simulink model "Rasmusson"  (Simulink 7.1)
settings: Solver=ode15s  StartTime=0.0  StopTime=500  FixedStep=1e-4  MaxStep=0.1  RelTol=1e-6
undefined symbols (not defined in the file): Acap, aKss, ato_f, ato_s, aur, C2, C3, C4, Cai, CaJSR, CaNSR, Cao, Cass, CK1, CK2, Cm, CMDN_tot, CNa1, CNa2, CSQN_tot, ECa_L, ECl, F, GCab, GCaL, GCl_Ca, GKr, GKs, GKss, GKtof, GKtos, GKur, GNa, GNab, HTRPN_tot, HTRPNCa, I1, I1Na, I2, I2Na, I3, ICaL_max, ICNa2, ICNa3, IFNa, IK, iKss, INaK_max, Ip_Ca_max, ito_f, ito_s, iur, ka1, ka2, kb, kb1, kb2, kc1, kc2, kf ... (+45)
(part 2 of 2)

== system Rasmusson/Concentrations/Caconcentration/Cafluxes/Jtrpn ==
  Add : Sum  Inputs=+-+-  OutDataType=sfix(16)  OutScaling=2^-10
  Divide : Product  Inputs=***  OutDataType=sfix(16)  OutScaling=2^-10
  Divide1 : Product  Inputs=**  OutDataType=sfix(16)  OutScaling=2^-10
  Divide2 : Product  Inputs=***  OutDataType=sfix(16)  OutScaling=2^-10
  Divide3 : Product  Inputs=**  OutDataType=sfix(16)  OutScaling=2^-10
  HTRPNtot : Constant  Value=HTRPN_tot  OutDataType=sfix(16)  OutScaling=2^0
  LTRPNtot : Constant  Value=LTRPN_tot  OutDataType=sfix(16)  OutScaling=2^0
  Subtract : Sum  Inputs=+-  OutDataType=sfix(16)  OutScaling=2^-10
  Subtract1 : Sum  Inputs=+-  OutDataType=sfix(16)  OutScaling=2^-10
  khtrpn+ : Constant  Value=khtrpn1  OutDataType=sfix(16)  OutScaling=2^0
  khtrpn- : Constant  Value=khtrpn2  OutDataType=sfix(16)  OutScaling=2^0
  kltrpn+ : Constant  Value=kltrpn1  OutDataType=sfix(16)  OutScaling=2^0
  kltrpn- : Constant  Value=kltrpn2  OutDataType=sfix(16)  OutScaling=2^0
  tag scope: Jtrpn=global
  wires:
  Add/1 -> [Jtrpn]
  Divide/1 -> Add/1
  khtrpn+/1 -> Divide/1
  [Cai] -> Divide/2, Divide2/2
  Subtract/1 -> Divide/3
  HTRPNtot/1 -> Subtract/1
  [HTRPNCa] -> Subtract/2, Divide1/2
  Divide1/1 -> Add/2
  khtrpn-/1 -> Divide1/1
  Divide2/1 -> Add/3
  kltrpn+/1 -> Divide2/1
  Subtract1/1 -> Divide2/3
  LTRPNtot/1 -> Subtract1/1
  [LTRPNCa] -> Subtract1/2, Divide3/2
  Divide3/1 -> Add/4
  kltrpn-/1 -> Divide3/1

== system Rasmusson/Concentrations/Caconcentration/Cafluxes/Jup ==
  Add : Sum  OutDataType=sfix(16)  OutScaling=2^-10
  Divide : Product  Inputs=**/  OutDataType=sfix(16)  OutScaling=2^-10
  Kmup : Constant  Value=Km_up  OutDataType=sfix(16)  OutScaling=2^0
  Product : Product  OutDataType=sfix(16)  OutScaling=2^0  RndMeth=Zero
  Product1 : Product  OutDataType=sfix(16)  OutScaling=2^0  RndMeth=Zero
  nu3 : Constant  Value=nu3  OutDataType=sfix(16)  OutScaling=2^0
  tag scope: Jup=global
  wires:
  Divide/1 -> [Jup]
  nu3/1 -> Divide/1
  [Cai] -> Product/1, Product/2
  Product/1 -> Divide/2, Add/1
  Add/1 -> Divide/3
  Kmup/1 -> Product1/1, Product1/2
  Product1/1 -> Add/2

== system Rasmusson/Concentrations/Caconcentration/Cafluxes/Jxfer ==
  Divide : Product  Inputs=*/  OutDataType=sfix(16)  OutScaling=2^-10
  Subtract : Sum  Inputs=+-  OutDataType=sfix(16)  OutScaling=2^-10
  tauxfer : Constant  Value=tauxfer  OutDataType=sfix(16)  OutScaling=2^0
  tag scope: Jxfer=global
  wires:
  Divide/1 -> [Jxfer]
  [Cass] -> Subtract/1
  [Cai] -> Subtract/2
  tauxfer/1 -> Divide/2
  Subtract/1 -> Divide/1

== system Rasmusson/Concentrations/Caconcentration/Cafluxes/PRyR ==
  Add : Sum  OutDataType=sfix(16)  OutScaling=2^-10
  Divide : Product  Inputs=**/  OutDataType=sfix(16)  OutScaling=2^-10
  Fcn : Fcn  Expr=exp(-(u-5)*(u-5)/648)
  Gain : Gain  Gain=-0.04  ParameterDataType=sfix(16)  ParameterScaling=2^0  OutDataType=sfix(16)  OutScaling=2^0
  Gain1 : Gain  Gain=-0.1  ParameterDataType=sfix(16)  ParameterScaling=2^0  OutDataType=sfix(16)  OutScaling=2^0
  ICaLmax : Constant  Value=ICaL_max  OutDataType=sfix(16)  OutScaling=2^0
  Integrator : Integrator  InitialConditionSource=external
  PRyR : Constant  Value=PRyR  OutDataType=sfix(16)  OutScaling=2^0
  tag scope: PRyR=global
  wires:
  Integrator/1 -> [PRyR], Gain/1
  Add/1 -> Integrator/1
  [ICAL] -> Divide/1
  Fcn/1 -> Divide/2
  ICaLmax/1 -> Divide/3
  [volt] -> Fcn/1
  Divide/1 -> Gain1/1
  Gain1/1 -> Add/2
  Gain/1 -> Add/1
  PRyR/1 -> Integrator/2

== system Rasmusson/Concentrations/Caconcentration/Ryanodine_receptors/PC1 ==
  Constant : Constant  OutDataType=sfix(16)  OutScaling=2^0
  Subtract : Sum  Inputs=+---  OutDataType=sfix(16)  OutScaling=2^-10
  tag scope: PC1=global
  wires:
  Subtract/1 -> [PC1]
  Constant/1 -> Subtract/1
  [PC2] -> Subtract/2
  [PO1] -> Subtract/3
  [PO2] -> Subtract/4

== system Rasmusson/Concentrations/Caconcentration/Ryanodine_receptors/PC2 ==
  Integrator : Integrator  InitialConditionSource=external  InitialCondition=0.16774e-3
  PC2 : Constant  Value=PC2  OutDataType=sfix(16)  OutScaling=2^0
  Product : Product  OutDataType=sfix(16)  OutScaling=2^0  RndMeth=Zero
  Product1 : Product  OutDataType=sfix(16)  OutScaling=2^0  RndMeth=Zero
  Subtract : Sum  Inputs=+-  OutDataType=sfix(16)  OutScaling=2^-10
  kc+ : Constant  Value=kc1  OutDataType=sfix(16)  OutScaling=2^0
  kc- : Constant  Value=kc2  OutDataType=sfix(16)  OutScaling=2^0
  tag scope: PC2=global
  wires:
  kc-/1 -> Product1/1
  kc+/1 -> Product/1
  Product1/1 -> Subtract/2
  Product/1 -> Subtract/1
  Integrator/1 -> Product1/2, [PC2]
  Subtract/1 -> Integrator/1
  [PO1] -> Product/2
  PC2/1 -> Integrator/2

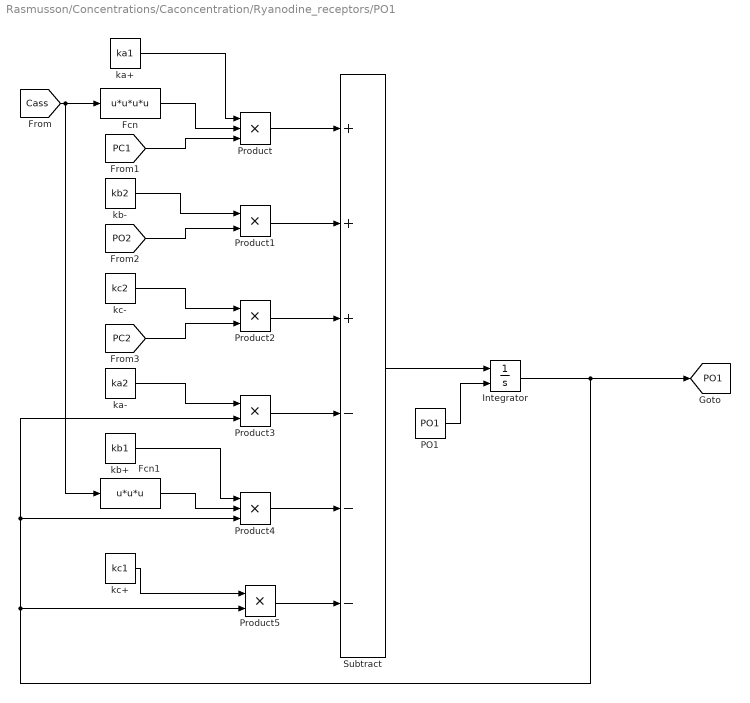
== system Rasmusson/Concentrations/Caconcentration/Ryanodine_receptors/PO1 ==
  Fcn : Fcn  Expr=u*u*u*u
  Fcn1 : Fcn  Expr=u*u*u
  Integrator : Integrator  InitialConditionSource=external  InitialCondition=0.149102e-4
  PO1 : Constant  Value=PO1  OutDataType=sfix(16)  OutScaling=2^0
  Product : Product  Inputs=3  OutDataType=sfix(16)  OutScaling=2^0  RndMeth=Zero
  Product{1..3,5} (4 alike) : Product  OutDataType=sfix(16)  OutScaling=2^0  RndMeth=Zero
  Product4 : Product  Inputs=3  OutDataType=sfix(16)  OutScaling=2^0  RndMeth=Zero
  Subtract : Sum  Inputs=+++---  OutDataType=sfix(16)  OutScaling=2^-10
  ka+ : Constant  Value=ka1  OutDataType=sfix(16)  OutScaling=2^0
  ka- : Constant  Value=ka2  OutDataType=sfix(16)  OutScaling=2^0
  kb+ : Constant  Value=kb1  OutDataType=sfix(16)  OutScaling=2^0
  kb- : Constant  Value=kb2  OutDataType=sfix(16)  OutScaling=2^0
  kc+ : Constant  Value=kc1  OutDataType=sfix(16)  OutScaling=2^0
  kc- : Constant  Value=kc2  OutDataType=sfix(16)  OutScaling=2^0
  tag scope: PO1=global
  wires:
  Subtract/1 -> Integrator/1
  [Cass] -> Fcn/1, Fcn1/1
  [PC1] -> Product/3
  Product/1 -> Subtract/1
  Product1/1 -> Subtract/2
  Product2/1 -> Subtract/3
  Product3/1 -> Subtract/4
  Product4/1 -> Subtract/5
  Product5/1 -> Subtract/6
  ka+/1 -> Product/1
  kb-/1 -> Product1/1
  [PO2] -> Product1/2
  kc-/1 -> Product2/1
  [PC2] -> Product2/2
  ka-/1 -> Product3/1
  kb+/1 -> Product4/1
  Fcn1/1 -> Product4/2
  kc+/1 -> Product5/1
  Fcn/1 -> Product/2
  Integrator/1 -> [PO1], Product3/2, Product4/3, Product5/2
  PO1/1 -> Integrator/2

== system Rasmusson/Concentrations/Caconcentration/Ryanodine_receptors/PO2 ==
  Fcn : Fcn  Expr=u*u*u
  Integrator : Integrator  InitialConditionSource=external  InitialCondition=0.951726e-10
  PO2 : Constant  Value=PO2  OutDataType=sfix(16)  OutScaling=2^0
  Product : Product  Inputs=3  OutDataType=sfix(16)  OutScaling=2^0  RndMeth=Zero
  Product1 : Product  OutDataType=sfix(16)  OutScaling=2^0  RndMeth=Zero
  Subtract : Sum  Inputs=+-  OutDataType=sfix(16)  OutScaling=2^-10
  kb+ : Constant  Value=kb1  OutDataType=sfix(16)  OutScaling=2^0
  kb- : Constant  Value=kb2  OutDataType=sfix(16)  OutScaling=2^0
  tag scope: PO2=global
  wires:
  Subtract/1 -> Integrator/1
  Integrator/1 -> [PO2], Product1/2
  Product/1 -> Subtract/1
  Product1/1 -> Subtract/2
  Fcn/1 -> Product/2
  kb+/1 -> Product/1
  [Cass] -> Fcn/1
  [PO1] -> Product/3
  kb-/1 -> Product1/1
  PO2/1 -> Integrator/2

== system Rasmusson/Ionic currents/ICaL/O/C1 ==
  Add : Sum  Inputs=+-------  OutDataType=sfix(16)  OutScaling=2^-10
  Constant : Constant  OutDataType=sfix(16)  OutScaling=2^0
  tag scope: C1=global
  wires:
  Add/1 -> [C1]
  Constant/1 -> Add/1
  [O] -> Add/2
  [C2] -> Add/3
  [C3] -> Add/4
  [C4] -> Add/5
  [I1] -> Add/6
  [I2] -> Add/7
  [I3] -> Add/8

== system Rasmusson/Ionic currents/ICaL/O/C2 ==
  Add : Sum  Inputs=++--  OutDataType=sfix(16)  OutScaling=2^-10
  C2 : Constant  Value=C2  OutDataType=sfix(16)  OutScaling=2^0
  Gain : Gain  Gain=4  ParameterDataType=sfix(16)  ParameterScaling=2^0  OutDataType=sfix(16)  OutScaling=2^0
  Gain1 : Gain  Gain=2  ParameterDataType=sfix(16)  ParameterScaling=2^0  OutDataType=sfix(16)  OutScaling=2^0
  Gain2 : Gain  Gain=3  ParameterDataType=sfix(16)  ParameterScaling=2^0  OutDataType=sfix(16)  OutScaling=2^0
  Integrator : Integrator  InitialConditionSource=external  InitialCondition=0.124216e-3
  Product{,1..3} (4 alike) : Product  OutDataType=sfix(16)  OutScaling=2^0  RndMeth=Zero
  tag scope: C2=global
  wires:
  Add/1 -> Integrator/1
  Gain/1 -> Add/1
  Product/1 -> Gain/1
  [alpha] -> Product/1, Product3/1
  [C1] -> Product/2
  [beta] -> Product1/1, Product2/1
  [C3] -> Product1/2
  Product1/1 -> Gain1/1
  Gain1/1 -> Add/2
  Product2/1 -> Add/3
  Integrator/1 -> [C2], Product2/2, Product3/2
  Product3/1 -> Gain2/1
  Gain2/1 -> Add/4
  C2/1 -> Integrator/2

== system Rasmusson/Ionic currents/ICaL/O/C3 ==
  Add : Sum  Inputs=++--  OutDataType=sfix(16)  OutScaling=2^-10
  C3 : Constant  Value=C3  OutDataType=sfix(16)  OutScaling=2^0
  Gain : Gain  Gain=3  ParameterDataType=sfix(16)  ParameterScaling=2^0  OutDataType=sfix(16)  OutScaling=2^0
  Gain1 : Gain  Gain=3  ParameterDataType=sfix(16)  ParameterScaling=2^0  OutDataType=sfix(16)  OutScaling=2^0
  Gain2 : Gain  Gain=2  ParameterDataType=sfix(16)  ParameterScaling=2^0  OutDataType=sfix(16)  OutScaling=2^0
  Gain3 : Gain  Gain=2  ParameterDataType=sfix(16)  ParameterScaling=2^0  OutDataType=sfix(16)  OutScaling=2^0
  Integrator : Integrator  InitialConditionSource=external  InitialCondition=0.578679e-8
  Product{,1..3} (4 alike) : Product  OutDataType=sfix(16)  OutScaling=2^0  RndMeth=Zero
  tag scope: C3=global
  wires:
  Add/1 -> Integrator/1
  Integrator/1 -> [C3], Product2/2, Product3/2
  Gain/1 -> Add/1
  Product/1 -> Gain/1
  [alpha] -> Product/1, Product3/1
  [C2] -> Product/2
  [beta] -> Product1/1, Product2/1
  [C4] -> Product1/2
  Product1/1 -> Gain1/1
  Gain1/1 -> Add/2
  Product2/1 -> Gain2/1
  Gain2/1 -> Add/3
  Product3/1 -> Gain3/1
  Gain3/1 -> Add/4
  C3/1 -> Integrator/2

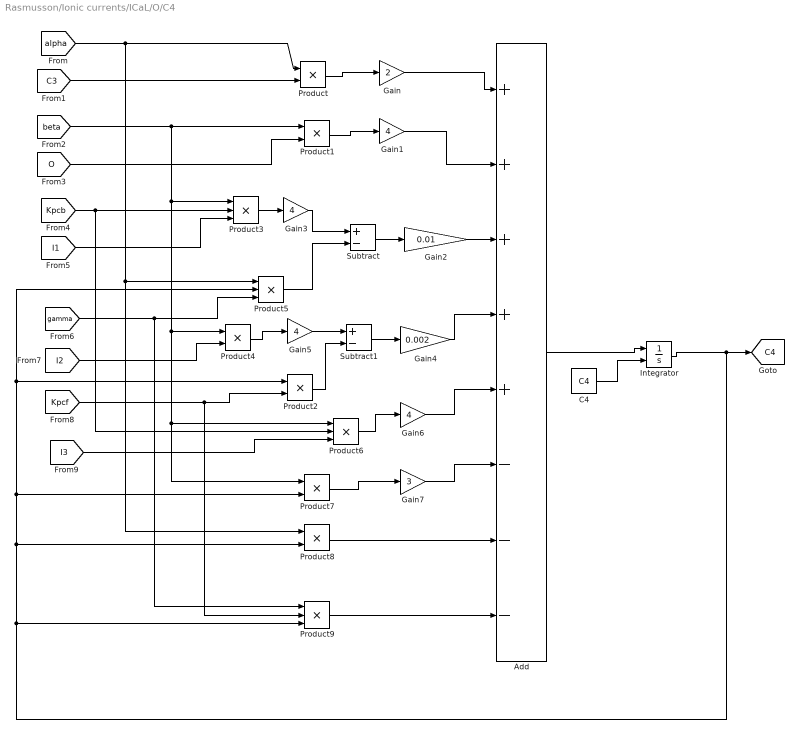
== system Rasmusson/Ionic currents/ICaL/O/C4 ==
  Add : Sum  Inputs=+++++---  OutDataType=sfix(16)  OutScaling=2^-10
  C4 : Constant  Value=C4  OutDataType=sfix(16)  OutScaling=2^0
  Gain : Gain  Gain=2  ParameterDataType=sfix(16)  ParameterScaling=2^0  OutDataType=sfix(16)  OutScaling=2^0
  Gain{1,3,5..6} (4 alike) : Gain  Gain=4  ParameterDataType=sfix(16)  ParameterScaling=2^0  OutDataType=sfix(16)  OutScaling=2^0
  Gain2 : Gain  Gain=0.01  ParameterDataType=sfix(16)  ParameterScaling=2^0  OutDataType=sfix(16)  OutScaling=2^0
  Gain4 : Gain  Gain=0.002  ParameterDataType=sfix(16)  ParameterScaling=2^0  OutDataType=sfix(16)  OutScaling=2^0
  Gain7 : Gain  Gain=3  ParameterDataType=sfix(16)  ParameterScaling=2^0  OutDataType=sfix(16)  OutScaling=2^0
  Integrator : Integrator  InitialConditionSource=external  InitialCondition=0.119816e-12
  Product{,1..2,4,7..8} (6 alike) : Product  OutDataType=sfix(16)  OutScaling=2^0  RndMeth=Zero
  Product{3,5..6,9} (4 alike) : Product  Inputs=3  OutDataType=sfix(16)  OutScaling=2^0  RndMeth=Zero
  Subtract : Sum  Inputs=+-  OutDataType=sfix(16)  OutScaling=2^-10
  Subtract1 : Sum  Inputs=+-  OutDataType=sfix(16)  OutScaling=2^-10
  tag scope: C4=global
  wires:
  Integrator/1 -> [C4], Product5/2, Product2/1, Product7/2, Product8/2, Product9/3
  Add/1 -> Integrator/1
  Gain/1 -> Add/1
  Product/1 -> Gain/1
  [alpha] -> Product/1, Product5/1, Product8/1
  [C3] -> Product/2
  Gain1/1 -> Add/2
  Product1/1 -> Gain1/1
  [beta] -> Product1/1, Product3/1, Product4/1, Product6/1, Product7/1
  [O] -> Product1/2
  Subtract/1 -> Gain2/1
  Gain2/1 -> Add/3
  Gain3/1 -> Subtract/1
  Product3/1 -> Gain3/1
  [Kpcb] -> Product3/2, Product6/2
  [I1] -> Product3/3
  Product5/1 -> Subtract/2
  [gamma] -> Product5/3, Product9/1
  Subtract1/1 -> Gain4/1
  Gain5/1 -> Subtract1/1
  Product4/1 -> Gain5/1
  [I2] -> Product4/2
  Product2/1 -> Subtract1/2
  [Kpcf] -> Product2/2, Product9/2
  Gain6/1 -> Add/5
  Product6/1 -> Gain6/1
  Gain4/1 -> Add/4
  [I3] -> Product6/3
  Gain7/1 -> Add/6
  Product7/1 -> Gain7/1
  Product8/1 -> Add/7
  Product9/1 -> Add/8
  C4/1 -> Integrator/2

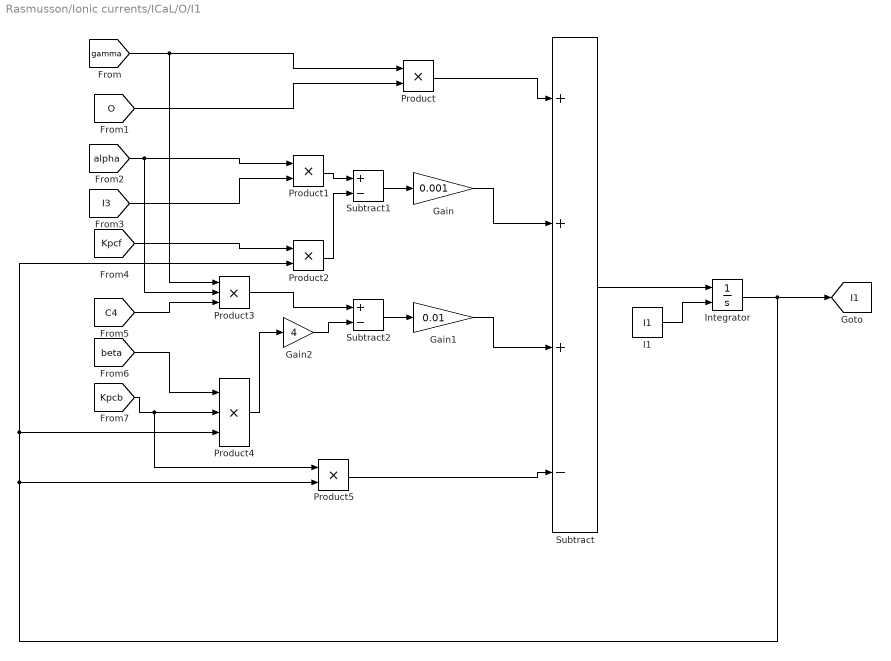
== system Rasmusson/Ionic currents/ICaL/O/I1 ==
  Gain : Gain  Gain=0.001  ParameterDataType=sfix(16)  ParameterScaling=2^0  OutDataType=sfix(16)  OutScaling=2^0
  Gain1 : Gain  Gain=0.01  ParameterDataType=sfix(16)  ParameterScaling=2^0  OutDataType=sfix(16)  OutScaling=2^0
  Gain2 : Gain  Gain=4  ParameterDataType=sfix(16)  ParameterScaling=2^0  OutDataType=sfix(16)  OutScaling=2^0
  I1 : Constant  Value=I1  OutDataType=sfix(16)  OutScaling=2^0
  Integrator : Integrator  InitialConditionSource=external  InitialCondition=0.497923e-18
  Product{,1..2,5} (4 alike) : Product  OutDataType=sfix(16)  OutScaling=2^0  RndMeth=Zero
  Product3 : Product  Inputs=3  OutDataType=sfix(16)  OutScaling=2^0  RndMeth=Zero
  Product4 : Product  Inputs=3  OutDataType=sfix(16)  OutScaling=2^0  RndMeth=Zero
  Subtract : Sum  Inputs=+++-  OutDataType=sfix(16)  OutScaling=2^-10
  Subtract1 : Sum  Inputs=+-  OutDataType=sfix(16)  OutScaling=2^-10
  Subtract2 : Sum  Inputs=+-  OutDataType=sfix(16)  OutScaling=2^-10
  tag scope: I1=global
  wires:
  Subtract/1 -> Integrator/1
  [gamma] -> Product/1, Product3/1
  [O] -> Product/2
  Product/1 -> Subtract/1
  Gain/1 -> Subtract/2
  Subtract1/1 -> Gain/1
  Integrator/1 -> [I1], Product2/2, Product4/3, Product5/2
  [alpha] -> Product1/1, Product3/2
  Product1/1 -> Subtract1/1
  Product2/1 -> Subtract1/2
  [I3] -> Product1/2
  [Kpcf] -> Product2/1
  Gain1/1 -> Subtract/3
  Subtract2/1 -> Gain1/1
  Gain2/1 -> Subtract2/2
  Product3/1 -> Subtract2/1
  Product4/1 -> Gain2/1
  [C4] -> Product3/3
  [beta] -> Product4/1
  [Kpcb] -> Product4/2, Product5/1
  Product5/1 -> Subtract/4
  I1/1 -> Integrator/2

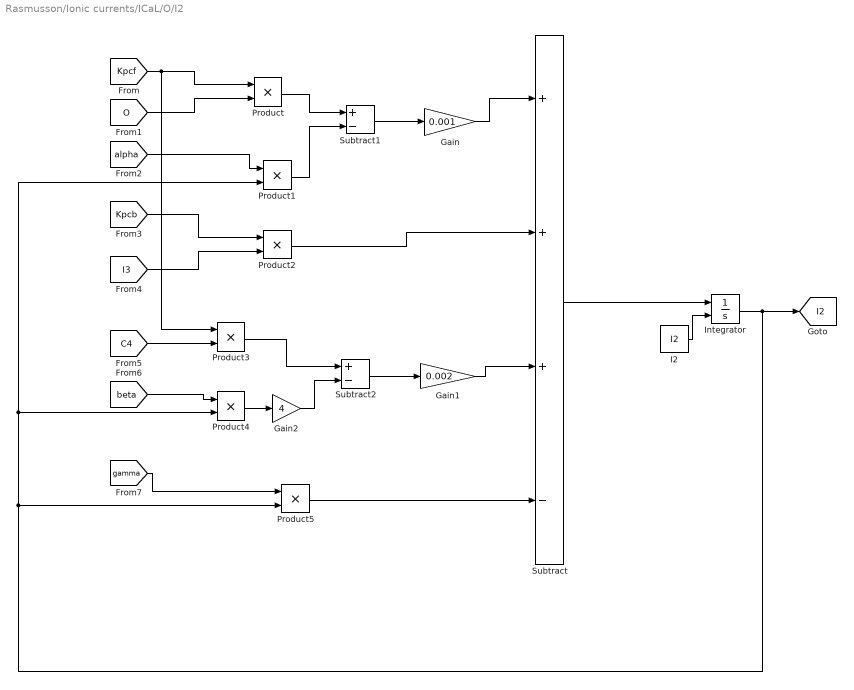
== system Rasmusson/Ionic currents/ICaL/O/I2 ==
  Gain : Gain  Gain=0.001  ParameterDataType=sfix(16)  ParameterScaling=2^0  OutDataType=sfix(16)  OutScaling=2^0
  Gain1 : Gain  Gain=0.002  ParameterDataType=sfix(16)  ParameterScaling=2^0  OutDataType=sfix(16)  OutScaling=2^0
  Gain2 : Gain  Gain=4  ParameterDataType=sfix(16)  ParameterScaling=2^0  OutDataType=sfix(16)  OutScaling=2^0
  I2 : Constant  Value=I2  OutDataType=sfix(16)  OutScaling=2^0
  Integrator : Integrator  InitialConditionSource=external  InitialCondition=0.345847e-13
  Product{,1..5} (6 alike) : Product  OutDataType=sfix(16)  OutScaling=2^0  RndMeth=Zero
  Subtract : Sum  Inputs=+++-  OutDataType=sfix(16)  OutScaling=2^-10
  Subtract1 : Sum  Inputs=+-  OutDataType=sfix(16)  OutScaling=2^-10
  Subtract2 : Sum  Inputs=+-  OutDataType=sfix(16)  OutScaling=2^-10
  tag scope: I2=global
  wires:
  Integrator/1 -> [I2], Product1/2, Product4/2, Product5/2
  Product1/1 -> Subtract1/2
  Product/1 -> Subtract1/1
  Subtract1/1 -> Gain/1
  [Kpcf] -> Product/1, Product3/1
  [O] -> Product/2
  [alpha] -> Product1/1
  Product2/1 -> Subtract/2
  [Kpcb] -> Product2/1
  [I3] -> Product2/2
  Product4/1 -> Gain2/1
  Gain2/1 -> Subtract2/2
  Subtract2/1 -> Gain1/1
  Product3/1 -> Subtract2/1
  [C4] -> Product3/2
  [beta] -> Product4/1
  [gamma] -> Product5/1
  Product5/1 -> Subtract/4
  Gain1/1 -> Subtract/3
  Gain/1 -> Subtract/1
  Subtract/1 -> Integrator/1
  I2/1 -> Integrator/2

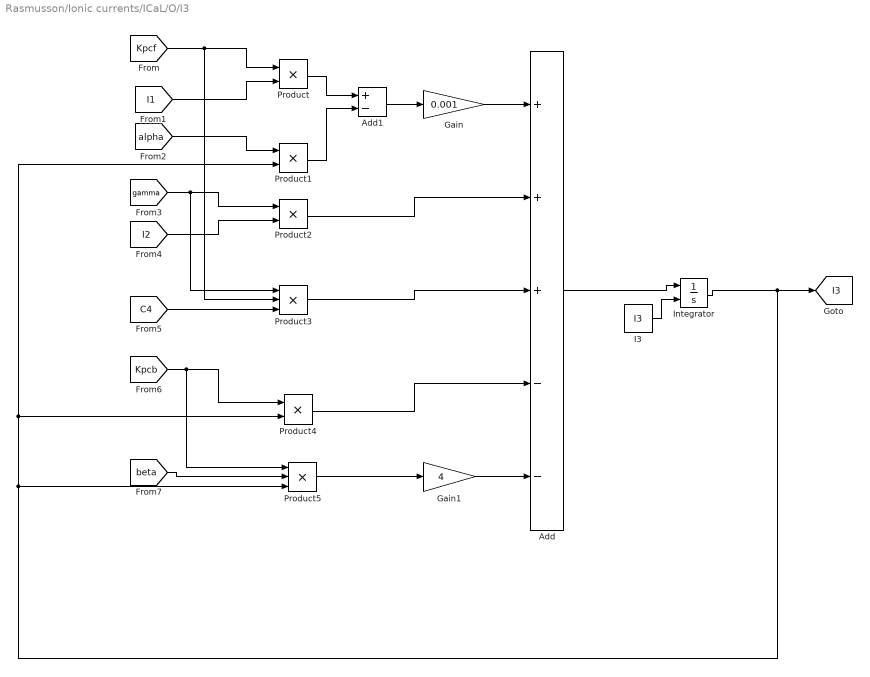
== system Rasmusson/Ionic currents/ICaL/O/I3 ==
  Add : Sum  Inputs=+++--  OutDataType=sfix(16)  OutScaling=2^-10
  Add1 : Sum  Inputs=+-  OutDataType=sfix(16)  OutScaling=2^-10
  Gain : Gain  Gain=0.001  ParameterDataType=sfix(16)  ParameterScaling=2^0  OutDataType=sfix(16)  OutScaling=2^0
  Gain1 : Gain  Gain=4  ParameterDataType=sfix(16)  ParameterScaling=2^0  OutDataType=sfix(16)  OutScaling=2^0
  I3 : Constant  Value=I3  OutDataType=sfix(16)  OutScaling=2^0
  Integrator : Integrator  InitialConditionSource=external  InitialCondition=0.185106e-13
  Product{,1..2,4} (4 alike) : Product  OutDataType=sfix(16)  OutScaling=2^0  RndMeth=Zero
  Product3 : Product  Inputs=3  OutDataType=sfix(16)  OutScaling=2^0  RndMeth=Zero
  Product5 : Product  Inputs=3  OutDataType=sfix(16)  OutScaling=2^0  RndMeth=Zero
  tag scope: I3=global
  wires:
  Integrator/1 -> [I3], Product1/2, Product4/2, Product5/3
  Add/1 -> Integrator/1
  Gain/1 -> Add/1
  Add1/1 -> Gain/1
  [alpha] -> Product1/1
  [I1] -> Product/2
  [Kpcf] -> Product/1, Product3/2
  Product/1 -> Add1/1
  Product1/1 -> Add1/2
  [gamma] -> Product2/1, Product3/1
  [I2] -> Product2/2
  Product2/1 -> Add/2
  Product3/1 -> Add/3
  [C4] -> Product3/3
  Product4/1 -> Add/4
  [Kpcb] -> Product4/1, Product5/1
  Gain1/1 -> Add/5
  Product5/1 -> Gain1/1
  [beta] -> Product5/2
  I3/1 -> Integrator/2

== system Rasmusson/Ionic currents/ICaL/O/Kpcb ==
  Kpcb : Constant  Value=Kpcb  OutDataType=sfix(16)  OutScaling=2^0
  tag scope: Kpcb=global
  wires:
  Kpcb/1 -> [Kpcb]

== system Rasmusson/Ionic currents/ICaL/O/Kpcf ==
  Kpcf : Fcn  Expr=13*(1-exp(-(u+14.5)*(u+14.5)/100))
  tag scope: Kpcf=global
  wires:
  [volt] -> Kpcf/1
  Kpcf/1 -> [Kpcf]

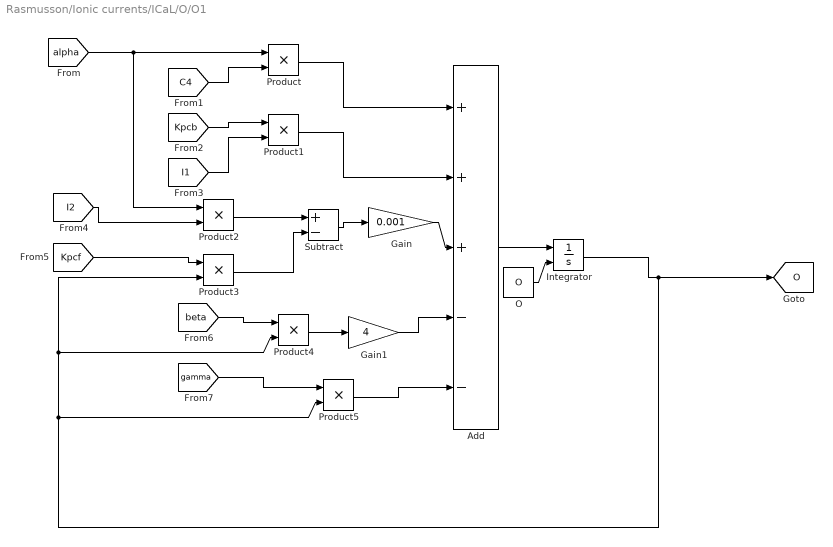
== system Rasmusson/Ionic currents/ICaL/O/O1 ==
  Add : Sum  Inputs=+++--  OutDataType=sfix(16)  OutScaling=2^-10
  Gain : Gain  Gain=0.001  ParameterDataType=sfix(16)  ParameterScaling=2^0  OutDataType=sfix(16)  OutScaling=2^0
  Gain1 : Gain  Gain=4  ParameterDataType=sfix(16)  ParameterScaling=2^0  OutDataType=sfix(16)  OutScaling=2^0
  Integrator : Integrator  InitialConditionSource=external  InitialCondition=0.930308e-18
  O : Constant  Value=O  OutDataType=sfix(16)  OutScaling=2^0
  Product{,1..5} (6 alike) : Product  OutDataType=sfix(16)  OutScaling=2^0  RndMeth=Zero
  Subtract : Sum  Inputs=+-  OutDataType=sfix(16)  OutScaling=2^-10
  tag scope: O=global
  wires:
  Add/1 -> Integrator/1
  Integrator/1 -> [O], Product3/2, Product4/2, Product5/2
  Product/1 -> Add/1
  [alpha] -> Product/1, Product2/1
  [C4] -> Product/2
  Product1/1 -> Add/2
  [Kpcb] -> Product1/1
  [I1] -> Product1/2
  Gain/1 -> Add/3
  Subtract/1 -> Gain/1
  Product2/1 -> Subtract/1
  Product3/1 -> Subtract/2
  [I2] -> Product2/2
  [Kpcf] -> Product3/1
  Gain1/1 -> Add/4
  Product4/1 -> Gain1/1
  [beta] -> Product4/1
  Product5/1 -> Add/5
  [gamma] -> Product5/1
  O/1 -> Integrator/2

== system Rasmusson/Ionic currents/ICaL/O/alpha ==
  alpha : Fcn  Expr=(0.4*exp((u+12)/10)*(1+0.7*exp(-(u+40)*(u+40)/10)-0.75*exp(-(u+20)*(u+20)/400)))/(1+0.12*exp((u+12)/10))
  tag scope: alpha=global
  wires:
  alpha/1 -> [alpha]
  [volt] -> alpha/1

== system Rasmusson/Ionic currents/ICaL/O/beta ==
  beta : Fcn  Expr=0.05*exp(-(u+12)/13)
  tag scope: beta=global
  wires:
  [volt] -> beta/1
  beta/1 -> [beta]

== system Rasmusson/Ionic currents/ICaL/O/gamma ==
  Divide : Product  Inputs=**/  OutDataType=sfix(16)  OutScaling=2^-10
  Kpchalf : Constant  Value=Kpc_half  OutDataType=sfix(16)  OutScaling=2^0
  Kpcmax : Constant  Value=Kpc_max  OutDataType=sfix(16)  OutScaling=2^0
  Subtract : Sum  OutDataType=sfix(16)  OutScaling=2^-10
  tag scope: gamma=global
  wires:
  Divide/1 -> [gamma]
  Kpcmax/1 -> Divide/1
  [Cass] -> Divide/2, Subtract/1
  Subtract/1 -> Divide/3
  Kpchalf/1 -> Subtract/2

== system Rasmusson/Ionic currents/INa/ONa/CNa1 ==
  Add : Sum  Inputs=+++---  OutDataType=sfix(16)  OutScaling=2^-10
  CNa1 : Constant  Value=CNa1  OutDataType=sfix(16)  OutScaling=2^0
  Integrator : Integrator  InitialConditionSource=external  InitialCondition=0.279132e-3
  Product{,1..5} (6 alike) : Product  OutDataType=sfix(16)  OutScaling=2^0  RndMeth=Zero
  tag scope: CNa1=global
  wires:
  [betaNa3] -> Product5/1
  [alphaNa13] -> Product4/1
  [betaNa12] -> Product3/1
  [IFNa] -> Product2/2
  [alphaNa3] -> Product2/1
  [ONa] -> Product1/2
  [betaNa13] -> Product1/1
  [CNa2] -> Product/2
  [alphaNa12] -> Product/1
  Product5/1 -> Add/6
  Product4/1 -> Add/5
  Product3/1 -> Add/4
  Product2/1 -> Add/3
  Product1/1 -> Add/2
  Product/1 -> Add/1
  Add/1 -> Integrator/1
  Integrator/1 -> Product5/2, Product4/2, Product3/2, [CNa1]
  CNa1/1 -> Integrator/2

== system Rasmusson/Ionic currents/INa/ONa/CNa2 ==
  Add : Sum  Inputs=+++---  OutDataType=sfix(16)  OutScaling=2^-10
  CNa2 : Constant  Value=CNa2  OutDataType=sfix(16)  OutScaling=2^0
  Integrator : Integrator  InitialConditionSource=external  InitialCondition=0.020752
  Product{,1..5} (6 alike) : Product  OutDataType=sfix(16)  OutScaling=2^0  RndMeth=Zero
  tag scope: CNa2=global
  wires:
  Integrator/1 -> [CNa2], Product3/2, Product4/2, Product5/2
  Add/1 -> Integrator/1
  Product/1 -> Add/1
  Product1/1 -> Add/2
  Product2/1 -> Add/3
  Product3/1 -> Add/4
  Product4/1 -> Add/5
  Product5/1 -> Add/6
  [alphaNa11] -> Product/1
  [CNa3] -> Product/2
  [betaNa12] -> Product1/1
  [CNa1] -> Product1/2
  [alphaNa3] -> Product2/1
  [ICNa2] -> Product2/2
  [betaNa11] -> Product3/1
  [alphaNa12] -> Product4/1
  [betaNa3] -> Product5/1
  CNa2/1 -> Integrator/2

== system Rasmusson/Ionic currents/INa/ONa/CNa3 ==
  Add : Sum  Inputs=+--------  OutDataType=sfix(16)  OutScaling=2^-10
  Constant : Constant  OutDataType=sfix(16)  OutScaling=2^0
  tag scope: CNa3=global
  wires:
  Add/1 -> [CNa3]
  Constant/1 -> Add/1
  [ONa] -> Add/2
  [CNa1] -> Add/3
  [CNa2] -> Add/4
  [IFNa] -> Add/5
  [I1Na] -> Add/6
  [I2Na] -> Add/7
  [ICNa2] -> Add/8
  [ICNa3] -> Add/9

== system Rasmusson/Ionic currents/INa/ONa/I1Na ==
  Add : Sum  Inputs=++--  OutDataType=sfix(16)  OutScaling=2^-10
  I1Na : Constant  Value=I1Na  OutDataType=sfix(16)  OutScaling=2^0
  Integrator : Integrator  InitialConditionSource=external  InitialCondition=0.673345e-6
  Product{,1,3,5} (4 alike) : Product  OutDataType=sfix(16)  OutScaling=2^0  RndMeth=Zero
  tag scope: I1Na=global
  wires:
  Product3/1 -> Add/3
  Product5/1 -> Add/4
  Integrator/1 -> Product5/2, Product3/2, [I1Na]
  Product/1 -> Add/1
  Product1/1 -> Add/2
  [alphaNa5] -> Product5/1
  [betaNa4] -> Product3/1
  [I2Na] -> Product1/2
  [betaNa5] -> Product1/1
  [IFNa] -> Product/2
  [alphaNa4] -> Product/1
  Add/1 -> Integrator/1
  I1Na/1 -> Integrator/2

== system Rasmusson/Ionic currents/INa/ONa/I2Na ==
  Add : Sum  Inputs=+-  OutDataType=sfix(16)  OutScaling=2^-10
  I2Na : Constant  Value=I2Na  OutDataType=sfix(16)  OutScaling=2^0
  Integrator : Integrator  InitialConditionSource=external  InitialCondition=0.155787e-8
  Product : Product  OutDataType=sfix(16)  OutScaling=2^0  RndMeth=Zero
  Product5 : Product  OutDataType=sfix(16)  OutScaling=2^0  RndMeth=Zero
  tag scope: I2Na=global
  wires:
  Add/1 -> Integrator/1
  [alphaNa5] -> Product/1
  [I1Na] -> Product/2
  [betaNa5] -> Product5/1
  Integrator/1 -> [I2Na], Product5/2
  Product5/1 -> Add/2
  Product/1 -> Add/1
  I2Na/1 -> Integrator/2

== system Rasmusson/Ionic currents/INa/ONa/ICNa2 ==
  Add : Sum  Inputs=+++---  OutDataType=sfix(16)  OutScaling=2^-10
  ICNa2 : Constant  Value=ICNa2  OutDataType=sfix(16)  OutScaling=2^0
  Integrator : Integrator  InitialConditionSource=external  InitialCondition=0.0113879
  Product{,1..5} (6 alike) : Product  OutDataType=sfix(16)  OutScaling=2^0  RndMeth=Zero
  tag scope: ICNa2=global
  wires:
  [alphaNa3] -> Product5/1
  [alphaNa12] -> Product4/1
  [betaNa11] -> Product3/1
  [CNa2] -> Product2/2
  [betaNa3] -> Product2/1
  [IFNa] -> Product1/2
  [betaNa12] -> Product1/1
  [ICNa3] -> Product/2
  [alphaNa11] -> Product/1
  Product5/1 -> Add/6
  Product4/1 -> Add/5
  Product3/1 -> Add/4
  Product2/1 -> Add/3
  Product1/1 -> Add/2
  Product/1 -> Add/1
  Add/1 -> Integrator/1
  Integrator/1 -> Product5/2, Product4/2, Product3/2, [ICNa2]
  ICNa2/1 -> Integrator/2

== system Rasmusson/Ionic currents/INa/ONa/ICNa3 ==
  Add : Sum  Inputs=++--  OutDataType=sfix(16)  OutScaling=2^-10
  ICNa3 : Constant  Value=ICNa3  OutDataType=sfix(16)  OutScaling=2^0
  Integrator : Integrator  InitialConditionSource=external  InitialCondition=0.342780
  Product{,1,3,5} (4 alike) : Product  OutDataType=sfix(16)  OutScaling=2^0  RndMeth=Zero
  tag scope: ICNa3=global
  wires:
  Add/1 -> Integrator/1
  [betaNa11] -> Product/1
  [ICNa2] -> Product/2
  [betaNa3] -> Product1/1
  [CNa3] -> Product1/2
  [alphaNa11] -> Product3/1
  [alphaNa3] -> Product5/1
  Product1/1 -> Add/2
  Product/1 -> Add/1
  Integrator/1 -> [ICNa3], Product3/2, Product5/2
  Product5/1 -> Add/4
  Product3/1 -> Add/3
  ICNa3/1 -> Integrator/2

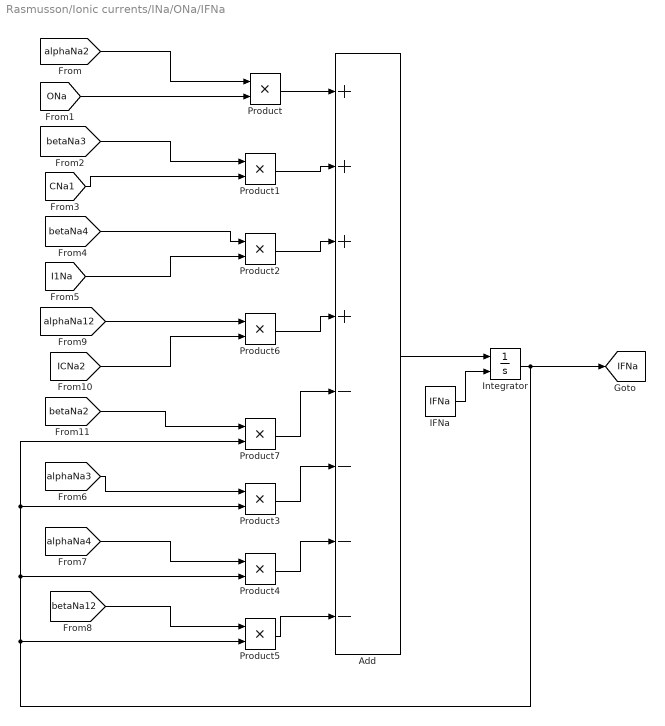
== system Rasmusson/Ionic currents/INa/ONa/IFNa ==
  Add : Sum  Inputs=++++----  OutDataType=sfix(16)  OutScaling=2^-10
  IFNa : Constant  Value=IFNa  OutDataType=sfix(16)  OutScaling=2^0
  Integrator : Integrator  InitialConditionSource=external  InitialCondition=0.153176e-3
  Product{,1..7} (8 alike) : Product  OutDataType=sfix(16)  OutScaling=2^0  RndMeth=Zero
  tag scope: IFNa=global
  wires:
  [betaNa12] -> Product5/1
  [alphaNa4] -> Product4/1
  [alphaNa3] -> Product3/1
  [I1Na] -> Product2/2
  [betaNa4] -> Product2/1
  [CNa1] -> Product1/2
  [betaNa3] -> Product1/1
  [ONa] -> Product/2
  [alphaNa2] -> Product/1
  Product2/1 -> Add/3
  Product1/1 -> Add/2
  Product/1 -> Add/1
  Add/1 -> Integrator/1
  Integrator/1 -> Product5/2, Product4/2, Product3/2, Product7/2, [IFNa]
  [ICNa2] -> Product6/2
  [alphaNa12] -> Product6/1
  Product6/1 -> Add/4
  [betaNa2] -> Product7/1
  Product7/1 -> Add/5
  Product3/1 -> Add/6
  Product4/1 -> Add/7
  Product5/1 -> Add/8
  IFNa/1 -> Integrator/2

== system Rasmusson/Ionic currents/INa/ONa/ONa ==
  Add : Sum  Inputs=++--  OutDataType=sfix(16)  OutScaling=2^-10
  Integrator : Integrator  InitialConditionSource=external  InitialCondition=0.713483e-6
  ONa : Constant  Value=ONa  OutDataType=sfix(16)  OutScaling=2^0
  Product{,1,3,5} (4 alike) : Product  OutDataType=sfix(16)  OutScaling=2^0  RndMeth=Zero
  tag scope: ONa=global
  wires:
  Add/1 -> Integrator/1
  [alphaNa13] -> Product/1
  [CNa1] -> Product/2
  [betaNa2] -> Product1/1
  [IFNa] -> Product1/2
  [betaNa13] -> Product3/1
  [alphaNa2] -> Product5/1
  Product1/1 -> Add/2
  Product/1 -> Add/1
  Integrator/1 -> [ONa], Product3/2, Product5/2
  Product5/1 -> Add/4
  Product3/1 -> Add/3
  ONa/1 -> Integrator/2

== system Rasmusson/Ionic currents/INa/ONa/alphaNa11 ==
  alphaNa11 : Fcn  Expr=3.802/(0.1027*exp(-(u+2.5)/17)+0.2*exp(-(u+2.5)/150))
  tag scope: alphaNa11=global
  wires:
  [volt] -> alphaNa11/1
  alphaNa11/1 -> [alphaNa11]

== system Rasmusson/Ionic currents/INa/ONa/alphaNa12 ==
  alphaNa12 : Fcn  Expr=3.802/(0.1027*exp(-(u+2.5)/15)+0.23*exp(-(u+2.5)/150))
  tag scope: alphaNa12=global
  wires:
  alphaNa12/1 -> [alphaNa12]
  [volt] -> alphaNa12/1

== system Rasmusson/Ionic currents/INa/ONa/alphaNa13 ==
  alphaNa13 : Fcn  Expr=3.802/(0.1027*exp(-(u+2.5)/12)+0.25*exp(-(u+2.5)/150))
  tag scope: alphaNa13=global
  wires:
  [volt] -> alphaNa13/1
  alphaNa13/1 -> [alphaNa13]

== system Rasmusson/Ionic currents/INa/ONa/alphaNa2 ==
  alphaNa2 : Fcn  Expr=1/(0.188495*exp(-(u+7)/16.6)+0.393956)
  tag scope: alphaNa2=global
  wires:
  alphaNa2/1 -> [alphaNa2]
  [volt] -> alphaNa2/1

== system Rasmusson/Ionic currents/INa/ONa/alphaNa3 ==
  alphaNa3 : Fcn  Expr=7e-7*exp(-(u+7)/7.7)
  tag scope: alphaNa3=global
  wires:
  alphaNa3/1 -> [alphaNa3]
  [volt] -> alphaNa3/1

== system Rasmusson/Ionic currents/INa/ONa/alphaNa4 ==
  Gain : Gain  Gain=0.001  ParameterDataType=sfix(16)  ParameterScaling=2^0  OutDataType=sfix(16)  OutScaling=2^0
  tag scope: alphaNa4=global
  wires:
  Gain/1 -> [alphaNa4]
  [alphaNa2] -> Gain/1

== system Rasmusson/Ionic currents/INa/ONa/alphaNa5 ==
  Constant : Constant  Value=95000  OutDataType=sfix(16)  OutScaling=2^0
  Divide : Product  Inputs=*/  OutDataType=sfix(16)  OutScaling=2^-10
  tag scope: alphaNa5=global
  wires:
  Divide/1 -> [alphaNa5]
  [alphaNa2] -> Divide/1
  Constant/1 -> Divide/2

== system Rasmusson/Ionic currents/INa/ONa/betaNa11 ==
  betaNa11 : Fcn  Expr=0.1917*exp(-(u+2.5)/20.3)
  tag scope: betaNa11=global
  wires:
  betaNa11/1 -> [betaNa11]
  [volt] -> betaNa11/1

== system Rasmusson/Ionic currents/INa/ONa/betaNa12 ==
  betaNa12 : Fcn  Expr=0.2*exp(-(u-2.5)/20.3)
  tag scope: betaNa12=global
  wires:
  [volt] -> betaNa12/1
  betaNa12/1 -> [betaNa12]

== system Rasmusson/Ionic currents/INa/ONa/betaNa13 ==
  betaNa13 : Fcn  Expr=0.22*exp(-(u-7.5)/20.3)
  tag scope: betaNa13=global
  wires:
  betaNa13/1 -> [betaNa13]
  [volt] -> betaNa13/1

== system Rasmusson/Ionic currents/INa/ONa/betaNa2 ==
  Divide : Product  Inputs=***//  OutDataType=sfix(16)  OutScaling=2^-10
  tag scope: betaNa2=global
  wires:
  Divide/1 -> [betaNa2]
  [alphaNa13] -> Divide/1
  [alphaNa2] -> Divide/2
  [alphaNa3] -> Divide/3
  [betaNa13] -> Divide/4
  [betaNa3] -> Divide/5

== system Rasmusson/Ionic currents/INa/ONa/betaNa3 ==
  betaNa3 : Fcn  Expr=0.0084+0.00002*(u+7)
  tag scope: betaNa3=global
  wires:
  [volt] -> betaNa3/1
  betaNa3/1 -> [betaNa3]

== system Rasmusson/Ionic currents/INa/ONa/betaNa4 ==
  tag scope: betaNa4=global
  wires:
  [alphaNa3] -> [betaNa4]

== system Rasmusson/Ionic currents/INa/ONa/betaNa5 ==
  Constant : Constant  Value=50  OutDataType=sfix(16)  OutScaling=2^0
  Divide : Product  Inputs=*/  OutDataType=sfix(16)  OutScaling=2^-10
  tag scope: betaNa5=global
  wires:
  Divide/1 -> [betaNa5]
  [alphaNa3] -> Divide/1
  Constant/1 -> Divide/2

== system Rasmusson/Ionic currents/INaK/fNaK/sigma ==
  Constant : Constant  OutDataType=sfix(16)  OutScaling=2^0
  Constant1 : Constant  Value=7  OutDataType=sfix(16)  OutScaling=2^0
  Constant2 : Constant  Value=67300  OutDataType=sfix(16)  OutScaling=2^0
  Divide : Product  Inputs=*/  OutDataType=sfix(16)  OutScaling=2^-10
  Divide1 : Product  Inputs=*/  OutDataType=sfix(16)  OutScaling=2^-10
  Math Function : Math  OutDataType=sfix(16)  OutScaling=2^0  SaturateOnIntegerOverflow=on
  Nao : Constant  Value=Nao  OutDataType=sfix(16)  OutScaling=2^0
  Subtract : Sum  Inputs=+-  OutDataType=sfix(16)  OutScaling=2^-10
  tag scope: sigma=global
  wires:
  Divide/1 -> [sigma]
  Constant1/1 -> Divide/2
  Subtract/1 -> Divide/1
  Constant/1 -> Subtract/2
  Math Function/1 -> Subtract/1
  Nao/1 -> Divide1/1
  Constant2/1 -> Divide1/2
  Divide1/1 -> Math Function/1
